simulink model "w2_1"  (R2021a)
settings: Solver=VariableStepAuto  StartTime=0.0  StopTime=10.0  RelTol=1e-3
settings Model: Creator=AVM  LastModifiedBy=AVM

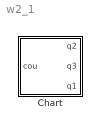
== system w2_1 ==
  Chart : Stateflow chart  TreatAsAtomicUnit=on

== stateflow chart w2_1/Chart ==
  state a_case5
    entry:
    q1=1;
    q2=0;
    q3=0;
  state a_case1
    entry:
    q1=0;
    q2=0;
    q3=0;
  state a000
    entry:
    q1=0;
    q2=0;
    q3=0;
  state a0004
    entry:
    q1=1;
    q2=0;
    q3=0;
  state a0001
    entry:
    q1=0;
    q2=0;
    q3=1;
  state a_case4
    entry:
    q1=0;
    q2=1;
    q3=1;
  state a_case2
    entry:
    q1=0;
    q2=0;
    q3=1;
  state a0003
    entry:
    q1=0;
    q2=1;
    q3=1;
  state a0002
    entry:
    q1=0;
    q2=1;
    q3=0;
  state a_case3
    entry:
    q1=0;
    q2=1;
    q3=0;
  (default) -> a000
  a_case5 -> a000 : [cou==1]
  a000 -> a_case1 : [cou==0]
  a0004 -> a_case5 : [cou==0]
  a_case1 -> a0001 : [cou==1]
  a_case4 -> a0004 : [cou==1]
  a0001 -> a_case2 : [cou==0]
  a0003 -> a_case4 : [cou==0]
  a_case2 -> a0002 : [cou==1]
  a_case3 -> a0003 : [cou==1]
  a0002 -> a_case3 : [cou==0]
  data: q2 output; q3 output; q1 output; cou input
